simulink model "modeloROBOTlinealisado"  (R2025a)
settings: Solver=VariableStepAuto  StartTime=0.0  StopTime=10.0  RelTol=1e-3
libraries: robotmaniplib x1
settings Model: Creator=Sandro  LastModifiedBy=Sandro

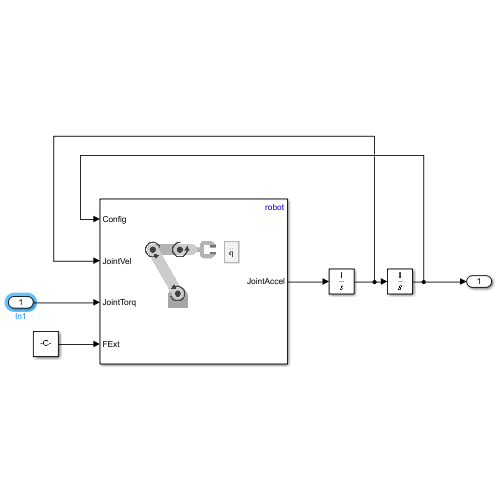
[thumbnail: Simulink's stored preview of the top-level diagram]
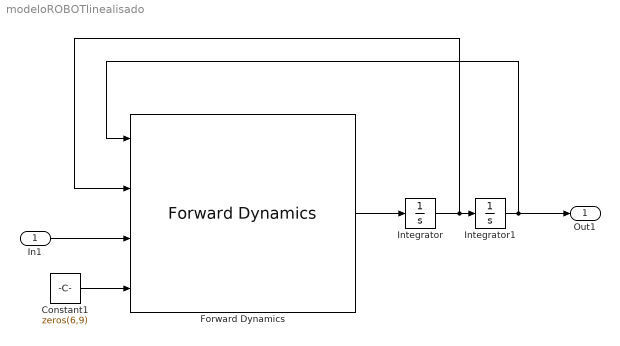
== system modeloROBOTlinealisado ==
  In1 : Inport  PortDimensions=6
  Constant1 : Constant  Value=zeros(6,9)
  Forward Dynamics : robotmaniplib/Forward Dynamics  RigidBodyTree=robot  SimulateUsing=Interpreted execution
  Integrator : Integrator
  Integrator1 : Integrator
  Out1 : Outport
  wires:
  Integrator/1 -> Forward Dynamics/2, Integrator1/1
  Forward Dynamics/1 -> Integrator/1
  Constant1/1 -> Forward Dynamics/4
  Integrator1/1 -> Out1/1, Forward Dynamics/1
  In1/1 -> Forward Dynamics/3
